simulink model "Model"  (R2021b)
settings: Solver=VariableStepAuto  StartTime=0.0  StopTime=SimTime  FixedStep=1  RelTol=1e-13  AbsTol=1e-13
values from neighbouring files (symbols this model uses):
  a = (39376)*1e3    (= 39376000)    [ScriptGroup20.m]
  alphaxy = (alphaxy/3)^2    (= 2.60887104e-10)    [ScriptGroup20.m]
  alphaz = (alphaz/3)^2    (= 3.75687767111e-08)    [ScriptGroup20.m]
  Aorthsens = 1e-3.*[1000,0.2,0.2;0.2,1000,0.2;0.2,0.2,1000]    [ScriptGroup20.m]
  burn_angle = deg2rad(30)    [ScriptGroup20.m]
  Controlled = 1    [ScriptGroup20.m]
  e = 0.7596    [ScriptGroup20.m]
  fgyro = 5    [ScriptGroup20.m]
  Fmax = 0.325/2    (= 0.1625)    [ScriptGroup20.m]
  fst = 5    [ScriptGroup20.m]
  hr0 = hrwslew(:,end)    [ScriptGroup20.m]
  i = deg2rad(28.4252)    [ScriptGroup20.m]
  I_tensor = I_unpacked    [ScriptGroup20.m]
  Iinv_tensor = inv(I_tensor)    [ScriptGroup20.m]
  Kdtrack = Kdtrack_track    (= 0.009)    [ScriptGroup20.m]
  Kpdet = 0.3    [ScriptGroup20.m]
  Kptrack = Kptrack_track    (= 0.009)    [ScriptGroup20.m]
  m_sc = factor*[1;1;1]    [ScriptGroup20.m]
  maxH = 50*1e-3    (= 0.05)    [ScriptGroup20.m]
  maxT = 8*1e-3    (= 0.008)    [ScriptGroup20.m]
  ModCont = 1    [ScriptGroup20.m]
  mu = 3.98600433e+5*1e9    (= 398600433000000)    [ScriptGroup20.m]
  normals = [n1,n2,n3,n4,n5,n6,n7,n8,n9,n10]    [ScriptGroup20.m]
  omega = deg2rad(0)    [ScriptGroup20.m]
  phi0 = Angtrueslew(1,1,end)    [ScriptGroup20.m]
  propmat = [rhos_sc;rhod_sc;rhos_sp;rhod_sp]    [ScriptGroup20.m]
  propsurf = [A1,A2,A3,A1,A2,A3,A7,A7,A9,A9]    [ScriptGroup20.m]
  psi0 = Angtrueslew(3,1,end)    [ScriptGroup20.m]
  r_cpTocm = [r1,r2,r3,r4,r5,r6,r7,r8,r9,r10]-ones(3,10).*cm    [ScriptGroup20.m]
  Re = 6371.01*1e3    (= 6371010)    [ScriptGroup20.m]
  sigma = deg2rad(0)    [ScriptGroup20.m]
  starcat = zeros(height(starcattab)-2,2)    [ScriptGroup20.m]
  T = R2*R1*[x*sin(gamma),-x*sin(gamma),x*sin(gamma),-x*sin(gamma);         -x*cos(gamma),l*sin(gamma),x*cos(gamma),-l*sin(gamma);         -l*sin(gamma),x*cos(gamma),l*sin(gamma),-x*cos(gamma)]    [ScriptGroup20.m]
  theta0 = Angtrueslew(2,1,end)    [ScriptGroup20.m]
  theta0orb = forbitslew(end)    [ScriptGroup20.m]
  thetb = thetb^2    [ScriptGroup20.m]
  thetn = thetn^2    [ScriptGroup20.m]
  thetsperc = 5*1e-4    (= 0.0005)    [ScriptGroup20.m]
  w = null(T)    [ScriptGroup20.m]
  w0_vector = wgyroslew(:,1,end)    [ScriptGroup20.m]
  w_lim = deg2rad(3)    [ScriptGroup20.m]
undefined symbols (not defined in the file or in its folder): DiscIntNeverNeededParam, phi_0, psi_0, theta_0
libraries: dspindex x22, matrix_library x20, vrlib x6, dspinverses x3, simulink_extras x3, dspfdesign x3, dspmtrx3 x2, simulink x1
(part 2 of 2)

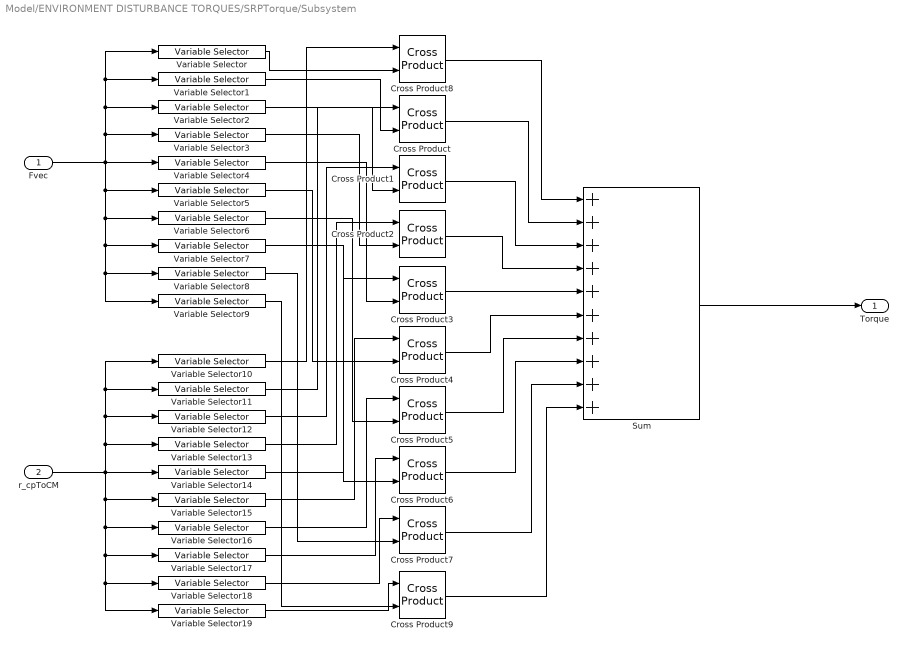
== system Model/ENVIRONMENT DISTURBANCE TORQUES/SRPTorque/Subsystem ==
  Fvec : Inport
  r_cpToCM : Inport  Port=2
  Cross Product{,1..9} (10 alike) : matrix_library/Cross Product
      settings: SourceProductBaseCode=SL
  Sum : Sum  Inputs=++++++++++
  Variable Selector : dspindex/Variable Selector  NumInputs=1  rowsOrCols=Columns  IdxMode=Fixed  Elements=[1]  ZerOneIdxMode=One-based  errmode=Clip Index  FillMode=on  FillValues=0
  Variable Selector1 : dspindex/Variable Selector  NumInputs=1  rowsOrCols=Columns  IdxMode=Fixed  Elements=[2]  ZerOneIdxMode=One-based  errmode=Clip Index  FillMode=on  FillValues=0
  Variable Selector10 : dspindex/Variable Selector  NumInputs=1  rowsOrCols=Columns  IdxMode=Fixed  Elements=[1]  ZerOneIdxMode=One-based  errmode=Clip Index  FillMode=on  FillValues=0
  Variable Selector11 : dspindex/Variable Selector  NumInputs=1  rowsOrCols=Columns  IdxMode=Fixed  Elements=[2]  ZerOneIdxMode=One-based  errmode=Clip Index  FillMode=on  FillValues=0
  Variable Selector12 : dspindex/Variable Selector  NumInputs=1  rowsOrCols=Columns  IdxMode=Fixed  Elements=[3]  ZerOneIdxMode=One-based  errmode=Clip Index  FillMode=on  FillValues=0
  Variable Selector13 : dspindex/Variable Selector  NumInputs=1  rowsOrCols=Columns  IdxMode=Fixed  Elements=[4]  ZerOneIdxMode=One-based  errmode=Clip Index  FillMode=on  FillValues=0
  Variable Selector14 : dspindex/Variable Selector  NumInputs=1  rowsOrCols=Columns  IdxMode=Fixed  Elements=[5]  ZerOneIdxMode=One-based  errmode=Clip Index  FillMode=on  FillValues=0
  Variable Selector15 : dspindex/Variable Selector  NumInputs=1  rowsOrCols=Columns  IdxMode=Fixed  Elements=[6]  ZerOneIdxMode=One-based  errmode=Clip Index  FillMode=on  FillValues=0
  Variable Selector16 : dspindex/Variable Selector  NumInputs=1  rowsOrCols=Columns  IdxMode=Fixed  Elements=[7]  ZerOneIdxMode=One-based  errmode=Clip Index  FillMode=on  FillValues=0
  Variable Selector17 : dspindex/Variable Selector  NumInputs=1  rowsOrCols=Columns  IdxMode=Fixed  Elements=[8]  ZerOneIdxMode=One-based  errmode=Clip Index  FillMode=on  FillValues=0
  Variable Selector18 : dspindex/Variable Selector  NumInputs=1  rowsOrCols=Columns  IdxMode=Fixed  Elements=[9]  ZerOneIdxMode=One-based  errmode=Clip Index  FillMode=on  FillValues=0
  Variable Selector19 : dspindex/Variable Selector  NumInputs=1  rowsOrCols=Columns  IdxMode=Fixed  Elements=[10]  ZerOneIdxMode=One-based  errmode=Clip Index  FillMode=on  FillValues=0
  Variable Selector2 : dspindex/Variable Selector  NumInputs=1  rowsOrCols=Columns  IdxMode=Fixed  Elements=[3]  ZerOneIdxMode=One-based  errmode=Clip Index  FillMode=on  FillValues=0
  Variable Selector3 : dspindex/Variable Selector  NumInputs=1  rowsOrCols=Columns  IdxMode=Fixed  Elements=[4]  ZerOneIdxMode=One-based  errmode=Clip Index  FillMode=on  FillValues=0
  Variable Selector4 : dspindex/Variable Selector  NumInputs=1  rowsOrCols=Columns  IdxMode=Fixed  Elements=[5]  ZerOneIdxMode=One-based  errmode=Clip Index  FillMode=on  FillValues=0
  Variable Selector5 : dspindex/Variable Selector  NumInputs=1  rowsOrCols=Columns  IdxMode=Fixed  Elements=[6]  ZerOneIdxMode=One-based  errmode=Clip Index  FillMode=on  FillValues=0
  Variable Selector6 : dspindex/Variable Selector  NumInputs=1  rowsOrCols=Columns  IdxMode=Fixed  Elements=[7]  ZerOneIdxMode=One-based  errmode=Clip Index  FillMode=on  FillValues=0
  Variable Selector7 : dspindex/Variable Selector  NumInputs=1  rowsOrCols=Columns  IdxMode=Fixed  Elements=[8]  ZerOneIdxMode=One-based  errmode=Clip Index  FillMode=on  FillValues=0
  Variable Selector8 : dspindex/Variable Selector  NumInputs=1  rowsOrCols=Columns  IdxMode=Fixed  Elements=[9]  ZerOneIdxMode=One-based  errmode=Clip Index  FillMode=on  FillValues=0
  Variable Selector9 : dspindex/Variable Selector  NumInputs=1  rowsOrCols=Columns  IdxMode=Fixed  Elements=[10]  ZerOneIdxMode=One-based  errmode=Clip Index  FillMode=on  FillValues=0
  Torque : Outport
  wires:
  Fvec/1 -> Variable Selector4/1, Variable Selector5/1, Variable Selector6/1, Variable Selector9/1, Variable Selector8/1, Variable Selector7/1, Variable Selector3/1, Variable Selector2/1, Variable Selector1/1, Variable Selector/1
  r_cpToCM/1 -> Variable Selector16/1, Variable Selector17/1, Variable Selector18/1, Variable Selector19/1, Variable Selector15/1, Variable Selector14/1, Variable Selector12/1, Variable Selector11/1, Variable Selector10/1, Variable Selector13/1
  Variable Selector10/1 -> Cross Product8/1
  Variable Selector11/1 -> Cross Product/1
  Variable Selector12/1 -> Cross Product1/1
  Variable Selector13/1 -> Cross Product2/1
  Variable Selector14/1 -> Cross Product3/1
  Variable Selector15/1 -> Cross Product4/1
  Variable Selector16/1 -> Cross Product5/1
  Variable Selector17/1 -> Cross Product6/1
  Variable Selector18/1 -> Cross Product7/1
  Variable Selector19/1 -> Cross Product9/1
  Variable Selector/1 -> Cross Product8/2
  Variable Selector1/1 -> Cross Product/2
  Variable Selector2/1 -> Cross Product1/2
  Variable Selector3/1 -> Cross Product2/2
  Variable Selector4/1 -> Cross Product3/2
  Variable Selector5/1 -> Cross Product4/2
  Variable Selector6/1 -> Cross Product5/2
  Variable Selector7/1 -> Cross Product6/2
  Variable Selector8/1 -> Cross Product7/2
  Variable Selector9/1 -> Cross Product9/2
  Cross Product3/1 -> Sum/5
  Cross Product2/1 -> Sum/4
  Cross Product1/1 -> Sum/3
  Cross Product/1 -> Sum/2
  Cross Product9/1 -> Sum/10
  Cross Product7/1 -> Sum/9
  Cross Product6/1 -> Sum/8
  Cross Product5/1 -> Sum/7
  Cross Product4/1 -> Sum/6
  Sum/1 -> Torque/1
  Cross Product8/1 -> Sum/1

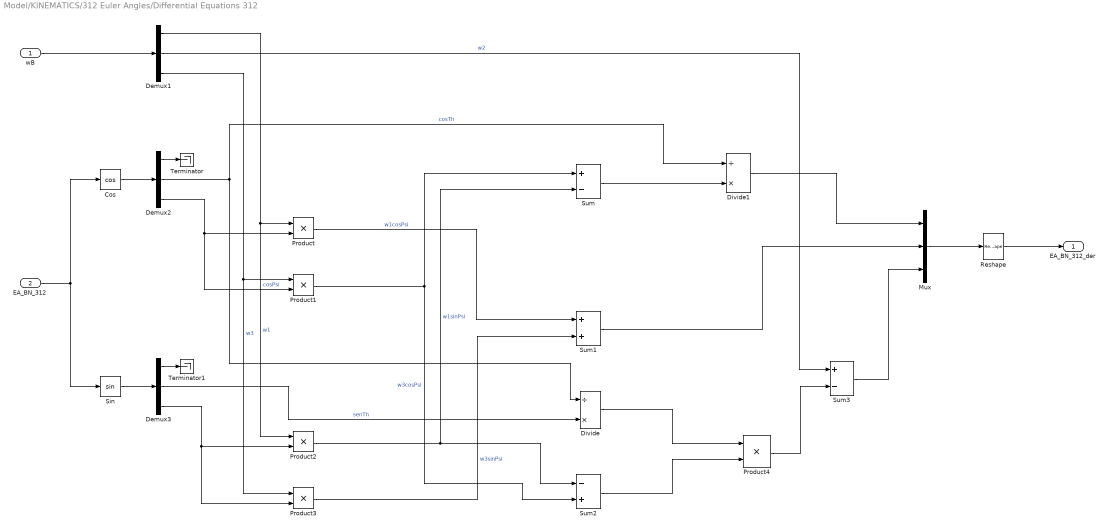
== system Model/KINEMATICS/312 Euler Angles/Differential Equations 312 ==
  wB : Inport
  EA_BN_312 : Inport  Port=2
  Cos : Trigonometry  Operator=cos
  Demux1 : Demux  Outputs=3
  Demux2 : Demux  Outputs=3
  Demux3 : Demux  Outputs=3
  Divide : Product  Inputs=/*
  Divide1 : Product  Inputs=/*
  Mux : Mux  Inputs=3
  Product{,1..4} (5 alike) : Product
  Reshape : Reshape  OutputDimensionality=Column vector (2-D)
  Sin : Trigonometry
  Sum : Sum  Inputs=+-
  Sum1 : Sum
  Sum2 : Sum  Inputs=-+
  Sum3 : Sum  Inputs=+-
  Terminator : Terminator
  Terminator1 : Terminator
  EA_BN_312_der : Outport
  wires:
  EA_BN_312/1 -> Cos/1, Sin/1
  wB/1 -> Demux1/1
  Cos/1 -> Demux2/1
  Sin/1 -> Demux3/1
  Demux2/1 -> Terminator/1
  Demux3/1 -> Terminator1/1
  Demux1/2 -> Sum3/1  "w2"
  Demux2/3 -> Product/2, Product1/2  "cosPsi"
  Demux1/1 -> Product2/1, Product/1  "w1"
  Demux1/3 -> Product3/1, Product1/1  "w3"
  Product/1 -> Sum1/1  "w1cosPsi"
  Product1/1 -> Sum2/2, Sum/1  "w3cosPsi"
  Demux2/2 -> Divide1/1, Divide/1  "cosTh"
  Demux3/2 -> Divide/2  "senTh"
  Product2/1 -> Sum2/1, Sum/2  "w1sinPsi"
  Product3/1 -> Sum1/2  "w3sinPsi"
  Demux3/3 -> Product2/2, Product3/2
  Sum1/1 -> Mux/2
  Sum/1 -> Divide1/2
  Divide1/1 -> Mux/1
  Divide/1 -> Product4/1
  Sum2/1 -> Product4/2
  Product4/1 -> Sum3/2
  Sum3/1 -> Mux/3
  Reshape/1 -> EA_BN_312_der/1
  Mux/1 -> Reshape/1

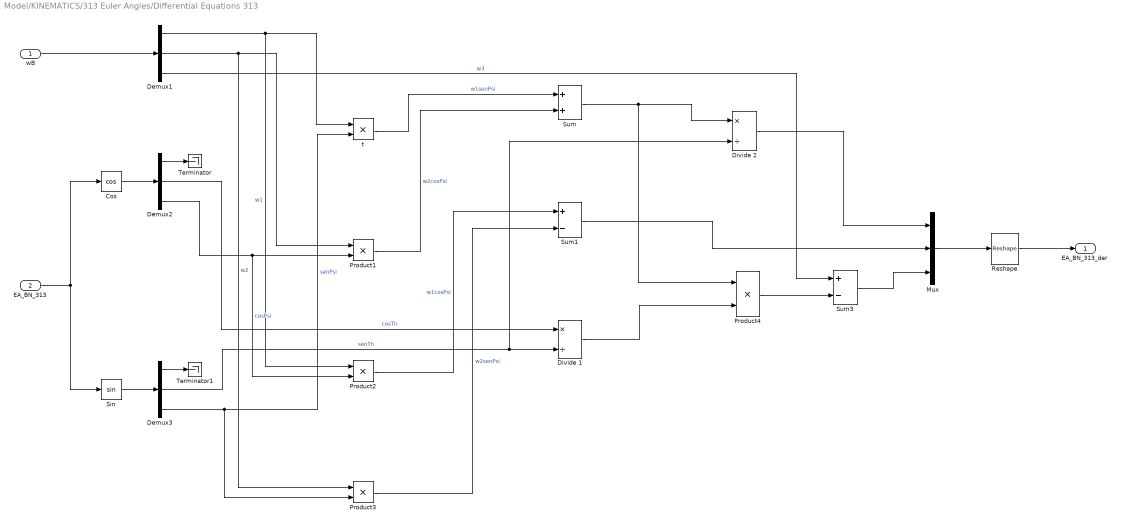
== system Model/KINEMATICS/313 Euler Angles/Differential Equations 313 ==
  wB : Inport
  EA_BN_313 : Inport  Port=2
  Cos : Trigonometry  Operator=cos
  Demux1 : Demux  Outputs=3
  Demux2 : Demux  Outputs=3
  Demux3 : Demux  Outputs=3
  Divide 1 : Product  Inputs=*/
  Divide 2 : Product  Inputs=*/
  Mux : Mux  Inputs=3
  Product{1..4} (4 alike) : Product
  Reshape : Reshape  OutputDimensionality=Column vector (2-D)
  Sin : Trigonometry
  Sum : Sum
  Sum1 : Sum  Inputs=+-
  Sum3 : Sum  Inputs=+-
  Terminator : Terminator
  Terminator1 : Terminator
  t : Product
  EA_BN_313_der : Outport
  wires:
  EA_BN_313/1 -> Cos/1, Sin/1
  wB/1 -> Demux1/1
  Mux/1 -> Reshape/1
  Cos/1 -> Demux2/1
  Sin/1 -> Demux3/1
  Demux1/1 -> Product2/1, t/1  "w1"
  Demux1/2 -> Product3/1, Product1/1  "w2"
  Demux1/3 -> Sum3/1  "w3"
  Demux2/1 -> Terminator/1
  Demux2/2 -> Divide 1/1  "cosTh"
  Demux2/3 -> Product2/2, Product1/2  "cosPsi"
  Demux3/1 -> Terminator1/1
  Demux3/2 -> Divide 2/2, Divide 1/2  "senTh"
  Demux3/3 -> t/2, Product3/2  "senPsi"
  t/1 -> Sum/1  "w1senPsi"
  Product1/1 -> Sum/2  "w2cosPsi"
  Product2/1 -> Sum1/1  "w1cosPsi"
  Product3/1 -> Sum1/2  "w2senPsi"
  Sum/1 -> Divide 2/1, Product4/1
  Divide 2/1 -> Mux/1
  Sum1/1 -> Mux/2
  Divide 1/1 -> Product4/2
  Product4/1 -> Sum3/2
  Sum3/1 -> Mux/3
  Reshape/1 -> EA_BN_313_der/1

== system Model/SENSORS/Gyro/ARW ==
  Mux : Mux  Inputs=3
  Random Number : RandomNumber  Variance=thetn  Seed=1  SampleTime=1/fgyro
  Random Number1 : RandomNumber  Variance=thetn  SampleTime=1/fgyro
  Random Number2 : RandomNumber  Variance=thetn  Seed=2  SampleTime=1/fgyro
  Out1 : Outport
  wires:
  Mux/1 -> Out1/1
  Random Number1/1 -> Mux/1
  Random Number2/1 -> Mux/3
  Random Number/1 -> Mux/2

== system Model/SENSORS/Gyro/Cscalefactor1 ==
  w : Inport
  Constant : Constant  Value=thetsperc
  Create Diagonal Matrix : dspmtrx3/Create Diagonal Matrix
      settings: SourceProductBaseCode=DS
  Demux : Demux  Outputs=3
  Identity Matrix : dspmtrx3/Identity Matrix  Inherit=off  N=3  Ts=1/fgyro  dataType=double  isSigned=on  wordLen=16  udDataType=sfix(16)  fracBitsMode=Best precision  numFracBits=15  OutDataTypeStr=double  LastOutDataTypeStr=double
  Mux : Mux  Inputs=3
  Product{,1..3} (4 alike) : Product
  Random Number : RandomNumber  SampleTime=1/fgyro
  Random Number1 : RandomNumber  Seed=1  SampleTime=1/fgyro
  Random Number2 : RandomNumber  Seed=2  SampleTime=1/fgyro
  Scope : Scope
  Sum : Sum
  C : Outport
  wires:
  Sum/1 -> C/1
  Create Diagonal Matrix/1 -> Sum/1
  Identity Matrix/1 -> Sum/2
  Mux/1 -> Create Diagonal Matrix/1
  w/1 -> Product3/1
  Constant/1 -> Product3/2
  Product3/1 -> Demux/1
  Random Number/1 -> Product/2
  Random Number1/1 -> Product1/2
  Random Number2/1 -> Product2/2
  Demux/3 -> Product2/1
  Demux/2 -> Product1/1
  Demux/1 -> Product/1
  Product2/1 -> Scope/1, Mux/3
  Product1/1 -> Mux/2
  Product/1 -> Mux/1

== system Model/SENSORS/Gyro/RRW ==
  Mux : Mux  Inputs=3
  Random Number : RandomNumber  Variance=thetb  SampleTime=1/fgyro
  Random Number1 : RandomNumber  Variance=thetb  Seed=1  SampleTime=1/fgyro
  Random Number2 : RandomNumber  Variance=thetb  Seed=2  SampleTime=1/fgyro
  Out1 : Outport
  wires:
  Mux/1 -> Out1/1
  Random Number2/1 -> Mux/3
  Random Number1/1 -> Mux/2
  Random Number/1 -> Mux/1

== system Model/SENSORS/StarCat/Error ==
  Sreal : Inport
  Lowpass Filter : dspfdesign/Lowpass Filter  FilterType=FIR  DesignForMinimumOrder=on  FilterOrder=50  PassbandFrequency=8e3  StopbandFrequency=12e3  PassbandRipple=0.1  StopbandAttenuation=80  InheritSampleRate=off  SampleRate=44100  SimulateUsing=Interpreted execution  roundingMode=Floor  coeffsDataTypeStr=fixdt(1,16)
  Lowpass Filter1 : dspfdesign/Lowpass Filter  FilterType=FIR  DesignForMinimumOrder=on  FilterOrder=50  PassbandFrequency=8e3  StopbandFrequency=12e3  PassbandRipple=0.1  StopbandAttenuation=80  InheritSampleRate=off  SampleRate=44100  SimulateUsing=Interpreted execution  roundingMode=Floor  coeffsDataTypeStr=fixdt(1,16)
  Lowpass Filter2 : dspfdesign/Lowpass Filter  FilterType=FIR  DesignForMinimumOrder=on  FilterOrder=50  PassbandFrequency=8e3  StopbandFrequency=12e3  PassbandRipple=0.1  StopbandAttenuation=80  InheritSampleRate=off  SampleRate=44100  SimulateUsing=Interpreted execution  roundingMode=Floor  coeffsDataTypeStr=fixdt(1,16)
  MATLAB Function : MATLAB Function  TreatAsAtomicUnit=on
  MATLAB Function1 : MATLAB Function  TreatAsAtomicUnit=on
  Random Number : RandomNumber  Variance=alphaxy  SampleTime=1/fst
  Random Number1 : RandomNumber  Variance=alphaz  Seed=2  SampleTime=1/fst
  Random Number2 : RandomNumber  Variance=alphaxy  Seed=1  SampleTime=1/fst
  Scope : Scope
  Scope1 : Scope
  Ssens : Outport
  wires:
  Lowpass Filter1/1 -> MATLAB Function/3(alphaz), Scope1/1
  MATLAB Function/1(Aeps) -> MATLAB Function1/1(Aeps), Scope/1
  Lowpass Filter/1 -> MATLAB Function/1(alphax)
  Random Number1/1 -> Lowpass Filter1/1
  Random Number/1 -> Lowpass Filter/1
  Lowpass Filter2/1 -> MATLAB Function/2(alphay)
  Random Number2/1 -> Lowpass Filter2/1
  Sreal/1 -> MATLAB Function1/2(Sreal)
  MATLAB Function1/1(Ssens) -> Ssens/1

== system Model/SENSORS/StarCat/rPolarisN ==
  Ra,Dec : Inport
  Cos : Trigonometry  Operator=cos
  Cos1 : Trigonometry  Operator=cos
  Degrees to Radians : simulink_extras/Transformations/Degrees to Radians
  Degrees to Radians1 : simulink_extras/Transformations/Degrees to Radians
  Matrix Concatenate : Concatenate  NumInputs=3  Mode=Multidimensional array  ConcatenateDimension=2
  Product : Product
  Product1 : Product
  Sin : Trigonometry
  Sin1 : Trigonometry
  Variable Selector : dspindex/Variable Selector  NumInputs=1  rowsOrCols=Columns  IdxMode=Fixed  Elements=1  ZerOneIdxMode=One-based  errmode=Clip Index  FillMode=on  FillValues=0
  Variable Selector1 : dspindex/Variable Selector  NumInputs=1  rowsOrCols=Columns  IdxMode=Fixed  Elements=1  ZerOneIdxMode=One-based  errmode=Clip Index  FillMode=on  FillValues=0
  rn : Outport
  wires:
  Degrees to Radians1/1 -> Sin/1, Cos/1
  Degrees to Radians/1 -> Sin1/1, Cos1/1
  Cos/1 -> Product1/1, Product/1
  Cos1/1 -> Product/2
  Sin1/1 -> Product1/2
  Variable Selector/1 -> Degrees to Radians/1
  Variable Selector1/1 -> Degrees to Radians1/1
  Ra,Dec/1 -> Variable Selector1/1, Variable Selector/1
  Product/1 -> Matrix Concatenate/1  "x"
  Product1/1 -> Matrix Concatenate/2  "y"
  Sin/1 -> Matrix Concatenate/3  "z"
  Matrix Concatenate/1 -> rn/1

== system Model/ACTUATORS/RW/RealRW/Desat ==
  Hr : Inport
  Abs : Abs
  Abs1 : Abs
  Constant : Constant  Value=maxH
  Constant1 : Constant  Value=maxT
  Delay : Delay  DelayLength=1
  Gain : Gain  Gain=-1
  GreaterThan : RelationalOperator  Operator=>  OutDataTypeStr=boolean  RndMeth=Simplest
  MATLAB Function : MATLAB Function  TreatAsAtomicUnit=on
  Max : MinMax  Function=max
  Max1 : MinMax  Function=max
  Product2 : Product
  Sign : Signum
  FlagDesat : Outport
  Mmotorsat : Outport  Port=2
  wires:
  Constant1/1 -> Product2/2
  Abs/1 -> GreaterThan/1
  Constant/1 -> GreaterThan/2
  Hr/1 -> Abs1/1, Sign/1, Abs/1
  Sign/1 -> Product2/1
  Gain/1 -> Mmotorsat/1
  Product2/1 -> Gain/1  "hrdot_desat"
  GreaterThan/1 -> Max1/1
  Max1/1 -> MATLAB Function/2(flaghr)
  Abs1/1 -> Max/1
  Delay/1 -> MATLAB Function/3(flagold)
  MATLAB Function/1(flag) -> FlagDesat/1, Delay/1
  Max/1 -> MATLAB Function/1(maxhr)

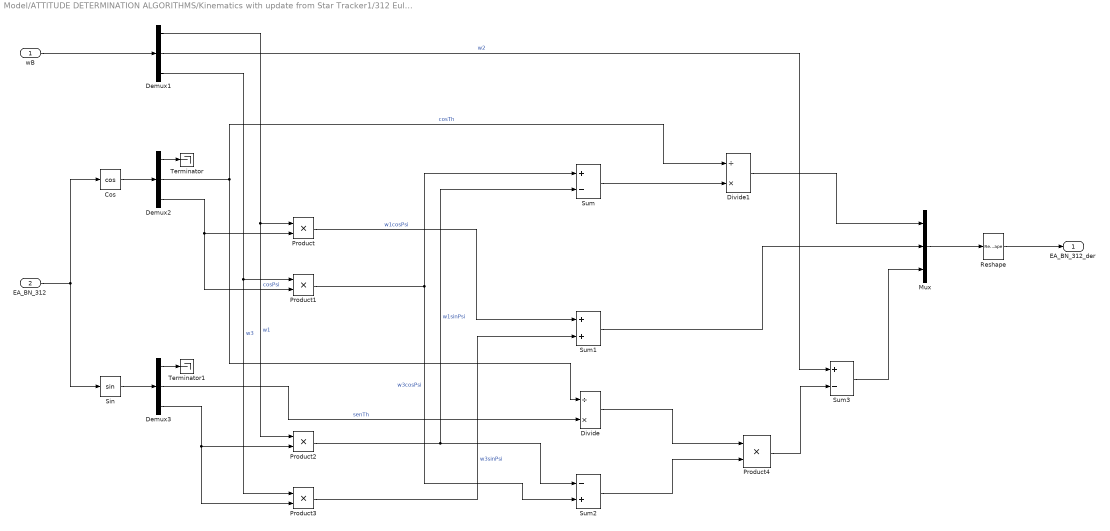
== system Model/ATTITUDE DETERMINATION ALGORITHMS/Kinematics with update from Star Tracker1/312 Euler Angles/Differential Equations 312 ==
  wB : Inport
  EA_BN_312 : Inport  Port=2
  Cos : Trigonometry  Operator=cos
  Demux1 : Demux  Outputs=3
  Demux2 : Demux  Outputs=3
  Demux3 : Demux  Outputs=3
  Divide : Product  Inputs=/*
  Divide1 : Product  Inputs=/*
  Mux : Mux  Inputs=3
  Product{,1..4} (5 alike) : Product
  Reshape : Reshape  OutputDimensionality=Column vector (2-D)
  Sin : Trigonometry
  Sum : Sum  Inputs=+-
  Sum1 : Sum
  Sum2 : Sum  Inputs=-+
  Sum3 : Sum  Inputs=+-
  Terminator : Terminator
  Terminator1 : Terminator
  EA_BN_312_der : Outport
  wires:
  Mux/1 -> Reshape/1
  Reshape/1 -> EA_BN_312_der/1
  Sum3/1 -> Mux/3
  Product4/1 -> Sum3/2
  Sum2/1 -> Product4/2
  Divide/1 -> Product4/1
  Divide1/1 -> Mux/1
  Sum/1 -> Divide1/2
  Sum1/1 -> Mux/2
  Demux3/3 -> Product3/2, Product2/2
  Product3/1 -> Sum1/2  "w3sinPsi"
  Product2/1 -> Sum/2, Sum2/1  "w1sinPsi"
  Demux3/2 -> Divide/2  "senTh"
  Demux2/2 -> Divide/1, Divide1/1  "cosTh"
  Product1/1 -> Sum/1, Sum2/2  "w3cosPsi"
  Product/1 -> Sum1/1  "w1cosPsi"
  Demux1/3 -> Product1/1, Product3/1  "w3"
  Demux1/1 -> Product/1, Product2/1  "w1"
  Demux2/3 -> Product1/2, Product/2  "cosPsi"
  Demux1/2 -> Sum3/1  "w2"
  Demux3/1 -> Terminator1/1
  Demux2/1 -> Terminator/1
  Sin/1 -> Demux3/1
  Cos/1 -> Demux2/1
  wB/1 -> Demux1/1
  EA_BN_312/1 -> Sin/1, Cos/1

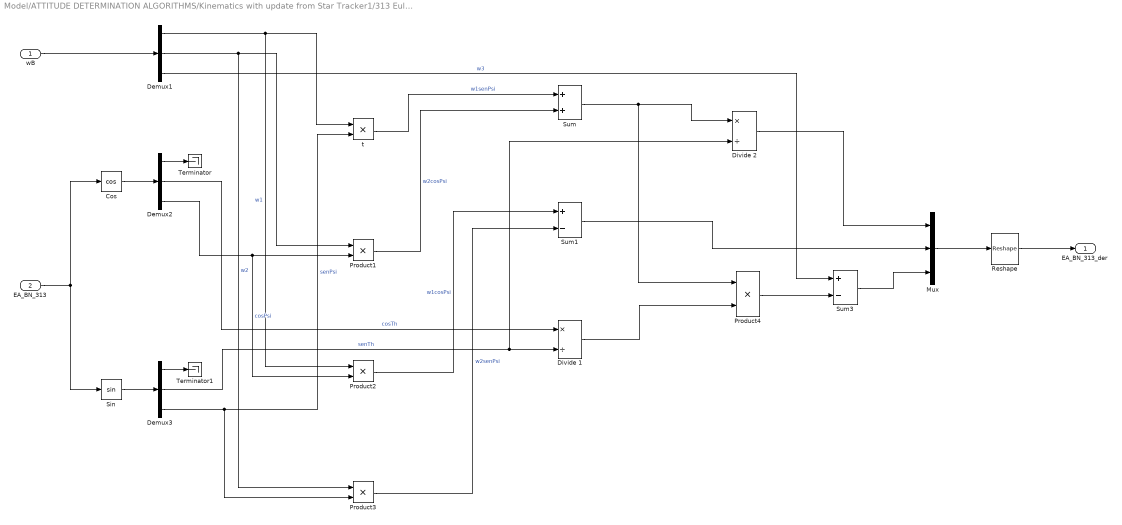
== system Model/ATTITUDE DETERMINATION ALGORITHMS/Kinematics with update from Star Tracker1/313 Euler Angles/Differential Equations 313 ==
  wB : Inport
  EA_BN_313 : Inport  Port=2
  Cos : Trigonometry  Operator=cos
  Demux1 : Demux  Outputs=3
  Demux2 : Demux  Outputs=3
  Demux3 : Demux  Outputs=3
  Divide 1 : Product  Inputs=*/
  Divide 2 : Product  Inputs=*/
  Mux : Mux  Inputs=3
  Product{1..4} (4 alike) : Product
  Reshape : Reshape  OutputDimensionality=Column vector (2-D)
  Sin : Trigonometry
  Sum : Sum
  Sum1 : Sum  Inputs=+-
  Sum3 : Sum  Inputs=+-
  Terminator : Terminator
  Terminator1 : Terminator
  t : Product
  EA_BN_313_der : Outport
  wires:
  Reshape/1 -> EA_BN_313_der/1
  Sum3/1 -> Mux/3
  Product4/1 -> Sum3/2
  Divide 1/1 -> Product4/2
  Sum1/1 -> Mux/2
  Divide 2/1 -> Mux/1
  Sum/1 -> Product4/1, Divide 2/1
  Product3/1 -> Sum1/2  "w2senPsi"
  Product2/1 -> Sum1/1  "w1cosPsi"
  Product1/1 -> Sum/2  "w2cosPsi"
  t/1 -> Sum/1  "w1senPsi"
  Demux3/3 -> Product3/2, t/2  "senPsi"
  Demux3/2 -> Divide 1/2, Divide 2/2  "senTh"
  Demux3/1 -> Terminator1/1
  Demux2/3 -> Product1/2, Product2/2  "cosPsi"
  Demux2/2 -> Divide 1/1  "cosTh"
  Demux2/1 -> Terminator/1
  Demux1/3 -> Sum3/1  "w3"
  Demux1/2 -> Product1/1, Product3/1  "w2"
  Demux1/1 -> t/1, Product2/1  "w1"
  Sin/1 -> Demux3/1
  Cos/1 -> Demux2/1
  Mux/1 -> Reshape/1
  wB/1 -> Demux1/1
  EA_BN_313/1 -> Sin/1, Cos/1

== matlab function Model/ATTITUDE DETERMINATION ALGORITHMS/SwitchAttitudeDetermination/SunPositionRespectN/MATLAB Function ==
  data: eps input; sn output; n_sun input; Rs input; time input
function sn = fcn(eps,n_sun,Rs,time)

eps=deg2rad(eps);

sn=Rs*[cos(n_sun*time);...
    sin(n_sun*time).*cos(eps);...
    sin(n_sun*time).*sin(eps)];


end

== matlab function Model/SENSORS/StarCat/Error/MATLAB Function ==
  data: alphax input; alphay input; Aeps output; alphaz input
function Aeps = fcn(alphax,alphay,alphaz)

Aeps=eye(3);
Aeps(1,2)=alphaz;
Aeps(1,3)=-alphay;
Aeps(2,1)=-alphaz;
Aeps(2,3)=alphax;
Aeps(3,1)=alphay;
Aeps(3,2)=-alphax;

end

== matlab function Model/SENSORS/StarCat/Error/MATLAB Function1 ==
  data: Aeps input; Ssens output; Sreal input
function Ssens = fcn(Aeps,Sreal)

[m,n]=size(Sreal);
Ssens=zeros(m,n);

Ssens(:,1:end)=Aeps*Sreal(:,1:end);


end

== matlab function Model/SENSORS/StarCat/MATLAB Function ==
  data: catrn input; Vn output; Abn input; num output
function [Vn,num] = fcn(catrn,Abn)

zvec=[Abn(3,1);Abn(3,2);Abn(3,3)];
angfov=deg2rad(20);
Vn=zeros(3,length(catrn));
num=0;


for i=1:length(catrn)
    if acos(dot(catrn(i,:),zvec))<angfov
        Vn(:,i)=catrn(i,:);
        num=num+1;
    end
    
end


end

== matlab function Model/CONTROL ALGORITHMS/Tracking/MATLAB Function ==
  data: matrix input; inversehat output
function inversehat = fcn(matrix)

inversehat=[0;0;0];

inversehat(1)=-matrix(2,3);
inversehat(2)=matrix(1,3);
inversehat(3)=-matrix(1,2);

end

== matlab function Model/ENVIRONMENT DISTURBANCE TORQUES/Gravity Gradient Torque/MATLAB Function ==
  data: I input; c input; M output; rnorm input
function M = fcn(I, c, rnorm)

mu=3.986*1e14;

c1=c(1);
c2=c(2);
c3=c(3);
I_x=I(1,1);
I_y=I(2,2);
I_z=I(3,3);

M=zeros(3,1);

M(1)=3*mu*(I_z-I_y)*c3*c2./rnorm.^3;
M(2)=3*mu*(I_x-I_z)*c1*c3./rnorm.^3;
M(3)=3*mu*(I_y-I_x)*c2*c1./rnorm.^3;

end

== matlab function Model/ENVIRONMENT DISTURBANCE TORQUES/MagneticTorque/MATLAB Function ==
  data: time input; mdir output
function mdir = fcn(time)

w_earth=729.2*1e-7;
ang=deg2rad(11.5);

mdir=zeros(3,1);

mdir(1)=sin(ang)*cos(w_earth*time);
mdir(2)=sin(ang)*sin(w_earth*time);
mdir(3)=cos(ang);

end

== matlab function Model/ENVIRONMENT DISTURBANCE TORQUES/OrbitRadialDirection/From N to eph ==
  data: sigma input; Aeph output; i input; omega input
function Aeph = fcn(sigma,i,omega)

R3sigma=[cos(sigma),sin(sigma),0;...
    -sin(sigma),cos(sigma),0;...
    0,0,1];
R1i=[1,0,0;...
    0,cos(i),sin(i);...
    0,-sin(i),cos(i)];
R3omega=[cos(omega),sin(omega),0;...
    -sin(omega),cos(omega),0;...
    0,0,1];

Aeph=R3omega*R1i*R3sigma;

end

== matlab function Model/ATTITUDE DETERMINATION ALGORITHMS/Kinematics with update from Star Tracker1/312 Euler Angles/Create DCM_BN_312 Matrix ==
  data: EA_BN_312 input; DCM_BN_312 output
function DCM_BN_312 = fcn(EA_BN_312)

DCM_BN_312 = zeros(3, 3);

DCM_BN_312(1,1) = cos(EA_BN_312(3))*cos(EA_BN_312(1)) - sin(EA_BN_312(3))*sin(EA_BN_312(1))*sin(EA_BN_312(2));
DCM_BN_312(1,2) = cos(EA_BN_312(3))*sin(EA_BN_312(1)) + sin(EA_BN_312(3))*cos(EA_BN_312(1))*sin(EA_BN_312(2));
DCM_BN_312(1,3) = -sin(EA_BN_312(3))*cos(EA_BN_312(2));
DCM_BN_312(2,1) = -sin(EA_BN_312(1))*cos(EA_BN_312(2));
DCM_BN_312(2,2) = cos(EA_BN_312(1))*cos(EA_BN_312(2));
DCM_BN_312(2,3) = sin(EA_BN_312(2));
DCM_BN_312(3,1) = sin(EA_BN_312(3))*cos(EA_BN_312(1)) + cos(EA_BN_312(3))*sin(EA_BN_312(1))*sin(EA_BN_312(2));
DCM_BN_312(3,2) = sin(EA_BN_312(3))*sin(EA_BN_312(1)) - cos(EA_BN_312(3))*cos(EA_BN_312(1))*sin(EA_BN_312(2));
DCM_BN_312(3,3) = cos(EA_BN_312(3))*cos(EA_BN_312(2));

end

== matlab function Model/ENVIRONMENT DISTURBANCE TORQUES/OrbitRadialDirection/From eph to rthetah ==
  data: Aeph input; Arthetah output; theta input
function Arthetah = fcn(Aeph,theta)

R3theta=[cos(theta),sin(theta),0;...
    -sin(theta),cos(theta),0;...
    0,0,1];

Arthetah=R3theta*Aeph;

end

== matlab function Model/ENVIRONMENT DISTURBANCE TORQUES/SRPTorque/MATLAB Function ==
  data: propmat input; propsurf input; Fvec output; sb input; normals input
function Fvec = fcn(propmat,propsurf,sb,normals)

%This script is already for a specific type of cubesat! I put every
%properties of spacecraft and solar panels toghether for not have too much
%disorder. Everytime you have to adapt the code.

P=1358/(3.*1e8);
n=normals;

%Computation forces

Fvec=zeros(3,10);

for i=1:(length(Fvec)-4)
    if dot(sb,n(:,i))>0
        Fvec(:,i)=-P*propsurf(i)*(dot(sb,n(:,i)))*((1-propmat(1)).*sb+...
            (2*propmat(1)*(dot(sb,n(:,i)))+(2/3)*propmat(2))*n(:,i));
    else
        Fvec(:,i)=[0;0;0];

    end
end

for i=(length(Fvec)-4):length(Fvec)
    if dot(sb,n(:,i))>0
        Fvec(:,i)=-P*propsurf(i)*(dot(sb,n(:,i)))*((1-propmat(3)).*sb+...
            (2*propmat(3)*(dot(sb,n(:,i)))+(2/3)*propmat(4))*n(:,i));
    else
        Fvec(:,i)=[0;0;0];

    end
end



end

== matlab function Model/ENVIRONMENT DISTURBANCE TORQUES/SunPositionRespectN/MATLAB Function ==
  data: eps input; sn output; n_sun input; Rs input; time input
function sn = fcn(eps,n_sun,Rs,time)

eps=deg2rad(eps);

sn=Rs*[cos(n_sun*time);...
    sin(n_sun*time).*cos(eps);...
    sin(n_sun*time).*sin(eps)];


end

== matlab function Model/KINEMATICS/312 Euler Angles/Create DCM_BN_312 Matrix ==
  data: EA_BN_312 input; DCM_BN_312 output
function DCM_BN_312 = fcn(EA_BN_312)

DCM_BN_312 = zeros(3, 3);

DCM_BN_312(1,1) = cos(EA_BN_312(3))*cos(EA_BN_312(1)) - sin(EA_BN_312(3))*sin(EA_BN_312(1))*sin(EA_BN_312(2));
DCM_BN_312(1,2) = cos(EA_BN_312(3))*sin(EA_BN_312(1)) + sin(EA_BN_312(3))*cos(EA_BN_312(1))*sin(EA_BN_312(2));
DCM_BN_312(1,3) = -sin(EA_BN_312(3))*cos(EA_BN_312(2));
DCM_BN_312(2,1) = -sin(EA_BN_312(1))*cos(EA_BN_312(2));
DCM_BN_312(2,2) = cos(EA_BN_312(1))*cos(EA_BN_312(2));
DCM_BN_312(2,3) = sin(EA_BN_312(2));
DCM_BN_312(3,1) = sin(EA_BN_312(3))*cos(EA_BN_312(1)) + cos(EA_BN_312(3))*sin(EA_BN_312(1))*sin(EA_BN_312(2));
DCM_BN_312(3,2) = sin(EA_BN_312(3))*sin(EA_BN_312(1)) - cos(EA_BN_312(3))*cos(EA_BN_312(1))*sin(EA_BN_312(2));
DCM_BN_312(3,3) = cos(EA_BN_312(3))*cos(EA_BN_312(2));

end

== matlab function Model/KINEMATICS/313 Euler Angles/Create DCM_BN_313 Matrix ==
  data: EA_BN_313 input; DCM_BN_313 output
function DCM_BN_313 = fcn(EA_BN_313)

DCM_BN_313 = zeros(3, 3);

DCM_BN_313(1,1) = cos(EA_BN_313(3))*cos(EA_BN_313(1)) - sin(EA_BN_313(3))*sin(EA_BN_313(1))*cos(EA_BN_313(2));
DCM_BN_313(1,2) = cos(EA_BN_313(3))*sin(EA_BN_313(1)) + sin(EA_BN_313(3))*cos(EA_BN_313(1))*cos(EA_BN_313(2));
DCM_BN_313(1,3) = sin(EA_BN_313(3))*sin(EA_BN_313(2));
DCM_BN_313(2,1) = - sin(EA_BN_313(3))*cos(EA_BN_313(1)) - cos(EA_BN_313(3))*sin(EA_BN_313(1))*cos(EA_BN_313(2));
DCM_BN_313(2,2) = - sin(EA_BN_313(3))*sin(EA_BN_313(1)) + cos(EA_BN_313(3))*cos(EA_BN_313(1))*cos(EA_BN_313(2));
DCM_BN_313(2,3) = cos(EA_BN_313(3))*sin(EA_BN_313(2));
DCM_BN_313(3,1) = sin(EA_BN_313(1))*sin(EA_BN_313(2));
DCM_BN_313(3,2) = - cos(EA_BN_313(1))*sin(EA_BN_313(2));
DCM_BN_313(3,3) = cos(EA_BN_313(2));


end

== matlab function Model/KINEMATICS/Factotum Switch ==
  data: DCM_BN input; flagIn input; IC_312 output; flagOut output; IC_313 output
function [IC_312, flagOut, IC_313] = fcn(DCM_BN, flagIn)
    
% estraggo i valori di theta
th312 = asin(DCM_BN(2,3));
th313 = acos(DCM_BN(3,3));

if flagIn == 1 

    if th312 < deg2rad(70) && th312 > deg2rad(-70)
        flagOut = 1;
    else
        flagOut = 0;
    end
    
else

    if th313 < deg2rad(160) && th313 > deg2rad(20)
        flagOut = 0;
    else
        flagOut = 1;
    end

end
    
% calcolo delle condizioni iniziali

th312_0 = asin(DCM_BN(2,3));
c_phi312_0 = DCM_BN(2,2)/cos(th312_0);
s_phi312_0 = - DCM_BN(2,1)/cos(th312_0);
phi312_0 = atan2(s_phi312_0, c_phi312_0);
c_psi312_0 = DCM_BN(3,3)/cos(th312_0);
s_psi312_0 = - DCM_BN(1,3)/cos(th312_0);
psi312_0 = atan2(s_psi312_0, c_psi312_0);

IC_312 = [phi312_0; th312_0; psi312_0];

if th313 == 0
    
    th313_0 = acos(DCM_BN(3,3)) + 1e-6;
    c_phi313_0 = - DCM_BN(3,2)/sin(th313_0);
    s_phi313_0 = DCM_BN(3,1)/sin(th313_0);
    phi313_0 = atan2(s_phi313_0, c_phi313_0);
    c_psi313_0 = DCM_BN(2,3)/sin(th313_0);
    s_psi313_0 = DCM_BN(1,3)/sin(th313_0);
    psi313_0 = atan2(s_psi313_0, c_psi313_0);

    IC_313 = [phi313_0; th313_0; psi313_0];

else

    th313_0 = acos(DCM_BN(3,3));
    c_phi313_0 = - DCM_BN(3,2)/sin(th313_0);
    s_phi313_0 = DCM_BN(3,1)/sin(th313_0);
    phi313_0 = atan2(s_phi313_0, c_phi313_0);
    c_psi313_0 = DCM_BN(2,3)/sin(th313_0);
    s_psi313_0 = DCM_BN(1,3)/sin(th313_0);
    psi313_0 = atan2(s_psi313_0, c_psi313_0);

    IC_313 = [phi313_0; th313_0; psi313_0];

end

end

== matlab function Model/KINEMATICS/Initial condition ==
  data: EA_BN_0 input; DCM_BN_0 output; flagIn_0 output
function [DCM_BN_0, flagIn_0] = fcn(EA_BN_0)

% estraggo gli angoli di eulero iniziali
phi_0 = EA_BN_0(1);
th_0 = EA_BN_0(2);
psi_0 = EA_BN_0(3);

if th_0 <= deg2rad(45) && th_0 >= deg2rad(-45) % integro con 312

    flagIn_0 = 1;

    DCM_BN_0 = [cos(psi_0)*cos(phi_0)-sin(psi_0)*sin(phi_0)*sin(th_0), cos(psi_0)*sin(phi_0)+sin(psi_0)*cos(phi_0)*sin(th_0), -sin(psi_0)*cos(th_0)
                -sin(phi_0)*cos(th_0), cos(phi_0)*cos(th_0), sin(th_0)
                sin(psi_0)*cos(phi_0)+cos(psi_0)*sin(phi_0)*sin(th_0), sin(psi_0)*sin(phi_0)-cos(psi_0)*cos(phi_0)*sin(th_0), cos(psi_0)*cos(th_0)];

else % integro con 313

    flagIn_0 = 0;

    DCM_BN_0 = [cos(psi_0)*cos(phi_0)-sin(psi_0)*sin(phi_0)*cos(th_0), cos(psi_0)*sin(phi_0)+sin(psi_0)*cos(phi_0)*cos(th_0), sin(psi_0)*sin(th_0)
                -sin(psi_0)*cos(phi_0)-cos(psi_0)*sin(phi_0)*cos(th_0), -sin(psi_0)*sin(phi_0)+cos(psi_0)*cos(phi_0)*cos(th_0), cos(psi_0)*sin(th_0)
                sin(phi_0)*sin(th_0), -cos(phi_0)*sin(th_0), cos(th_0)];

end

end

== matlab function Model/KINEMATICS/FinalConditions/MATLAB Function ==
  data: A0 input; Ang0 output
function Ang0 = fcn(A0)

DCM_BN=A0;

th312_0 = asin(DCM_BN(2,3));
c_phi312_0 = DCM_BN(2,2)/cos(th312_0);
s_phi312_0 = - DCM_BN(2,1)/cos(th312_0);
phi312_0 = atan2(s_phi312_0, c_phi312_0);
c_psi312_0 = DCM_BN(3,3)/cos(th312_0);
s_psi312_0 = - DCM_BN(1,3)/cos(th312_0);
psi312_0 = atan2(s_psi312_0, c_psi312_0);

Ang0=[phi312_0;th312_0;psi312_0];

end

== matlab function Model/ATTITUDE DETERMINATION ALGORITHMS/Kinematics with update from Star Tracker1/313 Euler Angles/Create DCM_BN_313 Matrix ==
  data: EA_BN_313 input; DCM_BN_313 output
function DCM_BN_313 = fcn(EA_BN_313)

DCM_BN_313 = zeros(3, 3);

DCM_BN_313(1,1) = cos(EA_BN_313(3))*cos(EA_BN_313(1)) - sin(EA_BN_313(3))*sin(EA_BN_313(1))*cos(EA_BN_313(2));
DCM_BN_313(1,2) = cos(EA_BN_313(3))*sin(EA_BN_313(1)) + sin(EA_BN_313(3))*cos(EA_BN_313(1))*cos(EA_BN_313(2));
DCM_BN_313(1,3) = sin(EA_BN_313(3))*sin(EA_BN_313(2));
DCM_BN_313(2,1) = - sin(EA_BN_313(3))*cos(EA_BN_313(1)) - cos(EA_BN_313(3))*sin(EA_BN_313(1))*cos(EA_BN_313(2));
DCM_BN_313(2,2) = - sin(EA_BN_313(3))*sin(EA_BN_313(1)) + cos(EA_BN_313(3))*cos(EA_BN_313(1))*cos(EA_BN_313(2));
DCM_BN_313(2,3) = cos(EA_BN_313(3))*sin(EA_BN_313(2));
DCM_BN_313(3,1) = sin(EA_BN_313(1))*sin(EA_BN_313(2));
DCM_BN_313(3,2) = - cos(EA_BN_313(1))*sin(EA_BN_313(2));
DCM_BN_313(3,3) = cos(EA_BN_313(2));


end

== matlab function Model/ATTITUDE DETERMINATION ALGORITHMS/Kinematics with update from Star Tracker1/Factotum Switch ==
  data: DCM_BN input; flagIn input; IC_312 output; flagOut output; IC_313 output
function [IC_312, flagOut, IC_313] = fcn(DCM_BN, flagIn)
    
% estraggo i valori di theta
th312 = asin(DCM_BN(2,3));
th313 = acos(DCM_BN(3,3));

if flagIn == 1 

    if th312 < deg2rad(70) && th312 > deg2rad(-70)
        flagOut = 1;
    else
        flagOut = 0;
    end
    
else

    if th313 < deg2rad(160) && th313 > deg2rad(20)
        flagOut = 0;
    else
        flagOut = 1;
    end

end
    
% calcolo delle condizioni iniziali

th312_0 = asin(DCM_BN(2,3));
c_phi312_0 = DCM_BN(2,2)/cos(th312_0);
s_phi312_0 = - DCM_BN(2,1)/cos(th312_0);
phi312_0 = atan2(s_phi312_0, c_phi312_0);
c_psi312_0 = DCM_BN(3,3)/cos(th312_0);
s_psi312_0 = - DCM_BN(1,3)/cos(th312_0);
psi312_0 = atan2(s_psi312_0, c_psi312_0);

IC_312 = [phi312_0; th312_0; psi312_0];

if th313 == 0
    
    th313_0 = acos(DCM_BN(3,3)) + 1e-6;
    c_phi313_0 = - DCM_BN(3,2)/sin(th313_0);
    s_phi313_0 = DCM_BN(3,1)/sin(th313_0);
    phi313_0 = atan2(s_phi313_0, c_phi313_0);
    c_psi313_0 = DCM_BN(2,3)/sin(th313_0);
    s_psi313_0 = DCM_BN(1,3)/sin(th313_0);
    psi313_0 = atan2(s_psi313_0, c_psi313_0);

    IC_313 = [phi313_0; th313_0; psi313_0];

else

    th313_0 = acos(DCM_BN(3,3));
    c_phi313_0 = - DCM_BN(3,2)/sin(th313_0);
    s_phi313_0 = DCM_BN(3,1)/sin(th313_0);
    phi313_0 = atan2(s_phi313_0, c_phi313_0);
    c_psi313_0 = DCM_BN(2,3)/sin(th313_0);
    s_psi313_0 = DCM_BN(1,3)/sin(th313_0);
    psi313_0 = atan2(s_psi313_0, c_psi313_0);

    IC_313 = [phi313_0; th313_0; psi313_0];

end

end

== matlab function Model/ATTITUDE DETERMINATION ALGORITHMS/Kinematics with update from Star Tracker1/Initial condition ==
  data: DCM_BN_star input; flagIn_0 output
function flagIn_0 = fcn(DCM_BN_star)

theta_star = asin(DCM_BN_star(2,3));

if theta_star <= pi/4 && theta_star >= -pi/4

    flagIn_0 = 1;

else

    flagIn_0 = 0;

end

end

== matlab function Model/ACTUATORS/RW/RealRW/Desat/MATLAB Function ==
  data: maxhr input; flaghr input; flag output; flagold input
function flag = fcn(maxhr,flaghr,flagold)

lim=10*1e-3;
flag=0;

if flaghr==1
    flag=1;
end

if flagold==1 && maxhr>lim
    flag=1;
elseif flagold==1 && maxhr<=lim
    flag=0;
end



end

== matlab function Model/DESIDERED ATTITUDE/From N to eph ==
  data: sigma input; Aeph output; i input; omega input
function Aeph = fcn(sigma,i,omega)

R3sigma=[cos(sigma),sin(sigma),0;...
    -sin(sigma),cos(sigma),0;...
    0,0,1];
R1i=[1,0,0;...
    0,cos(i),sin(i);...
    0,-sin(i),cos(i)];
R3omega=[cos(omega),sin(omega),0;...
    -sin(omega),cos(omega),0;...
    0,0,1];

Aeph=R3omega*R1i*R3sigma;

end

== matlab function Model/DESIDERED ATTITUDE/From eph to rthetah ==
  data: Aeph input; Arthetah output; theta input
function Arthetah = fcn(Aeph,theta)

R3theta=[cos(theta),sin(theta),0;...
    -sin(theta),cos(theta),0;...
    0,0,1];

Arthetah=R3theta*Aeph;

end

== matlab function Model/ATTITUDE DETERMINATION ALGORITHMS/Kinematics with update from Star Tracker1/MATLAB Function ==
  data: DCM_BN_star input; IC_312_in input; flag_in input; star_out input; IC_312_out output; flag_out output
function [IC_312_out, flag_out] = fcn(DCM_BN_star, IC_312_in, flag_in, star_out)

if star_out == 0

    th312_0 = asin(DCM_BN_star(2,3));
    c_phi312_0 = DCM_BN_star(2,2)/cos(th312_0);
    s_phi312_0 = - DCM_BN_star(2,1)/cos(th312_0);
    phi312_0 = atan2(s_phi312_0, c_phi312_0);
    c_psi312_0 = DCM_BN_star(3,3)/cos(th312_0);
    s_psi312_0 = - DCM_BN_star(1,3)/cos(th312_0);
    psi312_0 = atan2(s_psi312_0, c_psi312_0);

    IC_312_out = [phi312_0; th312_0; psi312_0];

    if flag_in == 1
        flag_out = 0;
    else
        flag_out = flag_in;
    end

else
    
    IC_312_out = IC_312_in;
    flag_out = flag_in;

end

end

== matlab function Model/ATTITUDE DETERMINATION ALGORITHMS/Kinematics with update from Star Tracker1/MATLAB Function1 ==
  data: star_out input; flag_in input; IC_313_in input; flag_out output; DCM_BN_star input; IC_313_out output
function [flag_out, IC_313_out] = fcn(star_out, flag_in, IC_313_in, DCM_BN_star)

if star_out == 0

    th313_0 = acos(DCM_BN_star(3,3));
    c_phi313_0 = - DCM_BN_star(3,2)/sin(th313_0);
    s_phi313_0 = DCM_BN_star(3,1)/sin(th313_0);
    phi313_0 = atan2(s_phi313_0, c_phi313_0);
    c_psi313_0 = DCM_BN_star(2,3)/sin(th313_0);
    s_psi313_0 = DCM_BN_star(1,3)/sin(th313_0);
    psi313_0 = atan2(s_psi313_0, c_psi313_0);

    IC_313_out = [phi313_0; th313_0; psi313_0];

    if flag_in == 0
        flag_out = 1;
    else
        flag_out = flag_in;
    end

else
    
    IC_313_out = IC_313_in;
    flag_out = flag_in;

end

end

== matlab function Model/ATTITUDE DETERMINATION ALGORITHMS/SwitchAttitudeDetermination/MATLAB Function ==
  data: wB_m input; cos_alpha input; star_out output; burn_angle input; w_lim input; FlagStars input
function star_out = fcn(wB_m, cos_alpha, burn_angle, w_lim, FlagStars)

cos_lim = cos(burn_angle);
w_norm = norm(wB_m);


if cos_alpha > cos_lim || w_norm > w_lim || FlagStars < 10

    star_out = 0;

else

    star_out = 1;

end

end
